simulink model "File4"  (Simulink 9.1)
settings: Solver=ode23t  StartTime=0.0  StopTime=2  FixedStep=1e-8  RelTol=1e-3
libraries: powerlib x4, simulink x3, re_lib x1
settings Model: Creator=asus  LastModifiedBy=asus
settings DataIOCC: SaveFormat=Dataset
settings OptimizationCC: LifeSpan=auto
settings DebuggingCC: UnderspecifiedInitializationDetection=Simplified  MergeDetectMultiDrivingBlocksExec=error  SFUnexpectedBacktrackingDiag=error  SFNoUnconditionalDefaultTransitionDiag=error  SFExecutionAtInitializationDiag=warning
settings HardwareCC: ProdBitPerPointer=64  ProdBitPerSizeT=64  ProdBitPerPtrDiffT=64  ProdLargestAtomicFloat=Float  ProdIntDivRoundTo=Zero  ProdEndianess=LittleEndian  ProdWordSize=64  ProdHWDeviceType=Intel->x86-64 (Windows64)
settings ModelReferenceCC: PropagateSignalLabelsOutOfModel=on
settings CodeAppCC: StateflowObjectComments=off
settings GRTTargetCC: TargetLangStandard=C99 (ISO)  CombineOutputUpdateFcns=on  GRTInterface=off
settings ConfigComp: CovMetricSettings=dwe  CovHtmlReporting=off  CovSaveCumulativeToWorkspaceVar=off  CovSaveSingleToWorkspaceVar=off  CovExternalEMLEnable=on

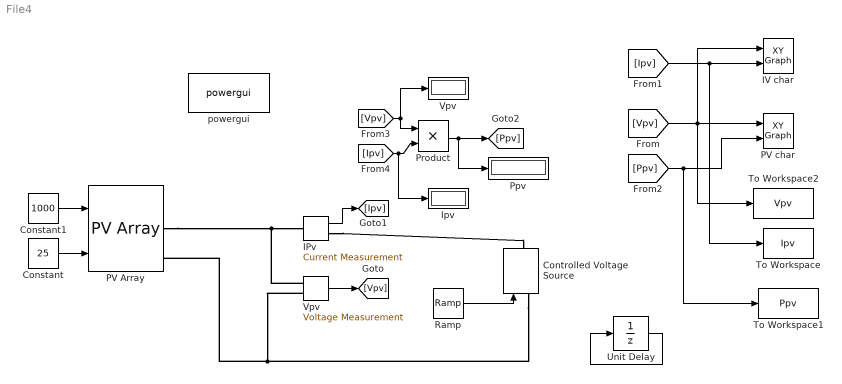
== system File4 ==
  " Ipv" : Display
  " Vpv" : Display
  Constant : Constant  Value=25
  Constant1 : Constant  Value=1000
  Controlled Voltage Source : powerlib/Electrical Sources/Controlled Voltage Source  Initialize=on  Source_Type=DC  Amplitude=0  Phase=0  Frequency=0  Measurements=None
  IPv : powerlib/Measurements/Current Measurement  PhasorSimulation=off  OutputType=Complex  PSBequivalent=0
  IV char : simulink/Sinks/XY Graph  xmin=0  xmax=230  ymin=0  ymax=12  st=1e-4
  PV Array : re_lib/Solar/PV Array  Npar=1  Nser=6  PlotType=array @ 1000 W/m2 & specified temperatures  S_vec="[ 1000  500  100 ]"  Temp_C_vec="[ 25  ]"  ModuleName=User-defined  PlotWhenSelected=off  Pm=249.9945  Ncell=60  Voc=36.54  Isc=9.44  Vm=30.45  Im=8.21  beta_Voc_pc=-0.32  alpha_Isc_pc=0.04  beta_Voc=-0.11693  alpha_Isc=0.003776  IL=9.4926  I0=6.8452e-11  nI=0.92814  Rsh=34.9757  Rs=0.19485  BAL=off  Tc=1e-6  Tfilter=5e-5
  PV char : simulink/Sinks/XY Graph  xmin=0  xmax=230  ymin=0  ymax=1600  st=1e-4
  Ppv : Display
  Product : Product
  Ramp : simulink/Sources/Ramp  slope=40*6  start=0  InitialOutput=0
  To Workspace : ToWorkspace  VariableName=Ipv  SaveFormat=Structure With Time  SampleTime=-1
  To Workspace1 : ToWorkspace  VariableName=Ppv  SaveFormat=Structure With Time  SampleTime=-1
  To Workspace2 : ToWorkspace  VariableName=Vpv  SaveFormat=Structure With Time  SampleTime=-1
  Unit Delay : UnitDelay  SampleTime=1e-6
  Vpv : powerlib/Measurements/Voltage Measurement  PhasorSimulation=off  OutputType=Complex  PSBequivalent=0
  powergui : powerlib/powergui  Priority=1  SimulationMode=Continuous  SampleTime=1e-8  frequency=60  Iterations=50  frequencyindice=0  Pbase=100e6  ErrMax=1e-4  UnitsV=kV  UnitsW=MW  buscounter=0  FunctionMessages=off  echomessages=off  EnableUseOfTLC=off  CurrentSourceSwitches=off  DisableSnubberDevices=off  DisableRonSwitches=off  DisableVfSwitches=off  DisplayEquations=off  SolverType=Tustin/Backward Euler (TBE)  Interpol=off  ExternalGateDelay=off  methode=off  Ts=100  x0status=blocks  SPID=on  SwTol=0  HookPort=off  RestoreLinks=warning  ResistiveCurrentMeasurement=off  Frange=[0:2:500]  Ylog=off  Xlog=on  ShowGrid=off  save=off  variable=ZData  structure=0  ZoomFFT=off  StartTime=0.0  cycles=1  DisplayStyle=1  fundamental=60  FreqAxis=off  MaxFrequency=1000  frequencyindicesteady=1  RmsSteady=1  display=off
  wires:
  Constant1/1 -> PV Array/1
  Constant/1 -> PV Array/2
  Ramp/1 -> Controlled Voltage Source/1
  Unit Delay/1 -> Unit Delay/1
  Vpv/1 -> [Vpv]
  IPv/1 -> [Ipv]
  Product/1 -> Ppv/1, [Ppv]
  [Vpv] -> Product/1, " Vpv"/1
  [Vpv] -> IV char/1, To Workspace2/1, PV char/1
  [Ipv] -> To Workspace/1, IV char/2
  [Ppv] -> To Workspace1/1, PV char/2
  [Ipv] -> " Ipv"/1, Product/2
  connections:
  PV Array/RConn1 -- Vpv/LConn1 -- IPv/LConn1
  Controlled Voltage Source/LConn1 -- Vpv/LConn2 -- PV Array/RConn2
  IPv/RConn1 -- Controlled Voltage Source/RConn1
